simulink model "Mostar"  (R2020a)
settings: Solver=ode45  StartTime=0  StopTime=4.5  FixedStep=0.01  RelTol=0.001  EnableMultiTasking=on
libraries: fmu_me_lib x2
settings Model: Creator=Tin Rabuzin  LastModifiedBy=meagh
settings DataIOCC: LimitDataPoints=on  SaveFormat=Array  ReturnWorkspaceOutputs=off  OutputSaveName=simout  OutputOption=SpecifiedOutputTimes  OutputTimes=[0:0.005:4.5]
settings OptimizationCC: ExpressionDepthLimit=2147483647  LifeSpan=inf
settings DebuggingCC: UnderspecifiedInitializationDetection=Classic  MergeDetectMultiDrivingBlocksExec=none  SolverPrmCheckMsg=warning  StateNameClashWarn=warning  SFUnexpectedBacktrackingDiag=warning  SFNoUnconditionalDefaultTransitionDiag=warning  SFExecutionAtInitializationDiag=none  ArithmeticOperatorsInVariantConditions=warning
settings HardwareCC: ProdBitPerPointer=32  ProdBitPerSizeT=32  ProdBitPerPtrDiffT=32  ProdLargestAtomicFloat=None  ProdIntDivRoundTo=Undefined  ProdEndianess=Unspecified  ProdWordSize=32  ProdHWDeviceType=32-bit Generic
settings ModelReferenceCC: PropagateSignalLabelsOutOfModel=off
settings SFSimCC: SimUseLocalCustomCode=off  CustomCodeUndefinedFunction=UseInterfaceOnly
settings RTWCC: RTWUseLocalCustomCode=off
settings CodeAppCC: StateflowObjectComments=on
settings GRTTargetCC: TargetLangStandard=C89/C90 (ANSI)
settings ConfigComp: CovMetricSettings=dw  CovHtmlReporting=on  CovSaveCumulativeToWorkspaceVar=on  CovSaveSingleToWorkspaceVar=on  CovExternalEMLEnable=off

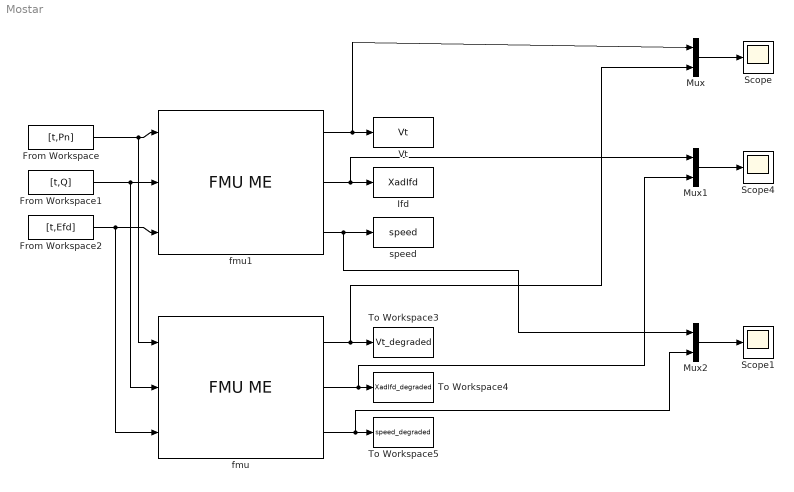
== system Mostar ==
  From Workspace : FromWorkspace  VariableName=[t,Pn]
  From Workspace1 : FromWorkspace  VariableName=[t,Q]
  From Workspace2 : FromWorkspace  VariableName=[t,Efd]
  Ifd : ToWorkspace  VariableName=XadIfd  SaveFormat=Structure With Time  SampleTime=0.005
  Mux : Mux  Inputs=2
  Mux1 : Mux  Inputs=2
  Mux2 : Mux  Inputs=2
  Scope : Scope
  Scope1 : Scope
  Scope4 : Scope
  To Workspace3 : ToWorkspace  VariableName=Vt_degraded  SaveFormat=Structure With Time  SampleTime=0.005
  To Workspace4 : ToWorkspace  VariableName=XadIfd_degraded  SaveFormat=Structure With Time  SampleTime=0.005
  To Workspace5 : ToWorkspace  VariableName=speed_degraded  SaveFormat=Structure With Time  SampleTime=0.005
  Vt : ToWorkspace  VariableName=Vt  SaveFormat=Structure With Time  SampleTime=0.005
  fmu : fmu_me_lib/FMU ME  Description=Simulates an FMU for Model Exchange 1.0 or Model Exchange 2.0.  dummy=0
  fmu1 : fmu_me_lib/FMU ME  Description=Simulates an FMU for Model Exchange 1.0 or Model Exchange 2.0.  dummy=0
  speed : ToWorkspace  VariableName=speed  SaveFormat=Structure With Time  SampleTime=0.005
  wires:
  fmu1/1 -> Mux/1, Vt/1
  From Workspace/1 -> fmu/1, fmu1/1
  From Workspace1/1 -> fmu/2, fmu1/2
  From Workspace2/1 -> fmu/3, fmu1/3
  fmu1/2 -> Mux1/1, Ifd/1
  fmu1/3 -> Mux2/1, speed/1
  fmu/1 -> Mux/2, To Workspace3/1
  fmu/3 -> Mux2/2, To Workspace5/1
  fmu/2 -> Mux1/2, To Workspace4/1
  Mux/1 -> Scope/1
  Mux1/1 -> Scope4/1
  Mux2/1 -> Scope1/1
